simulink model "sistema_fisico_completo"  (R2023b)
settings: Solver=FixedStepAuto  StartTime=0.0  StopTime=10.0  FixedStep=0.001  RelTol=1e-3
settings Model: Creator=Ferran  LastModifiedBy=Ferran
settings DebuggingCC: AlgebraicLoopMsg=none  ArtificialAlgebraicLoopMsg=none
settings ModelReferenceCC: ModelReferenceMinAlgLoopOccurrences=on

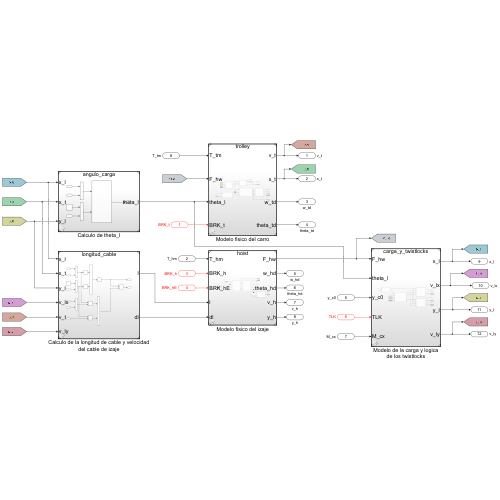
[thumbnail: Simulink's stored preview of the top-level diagram]
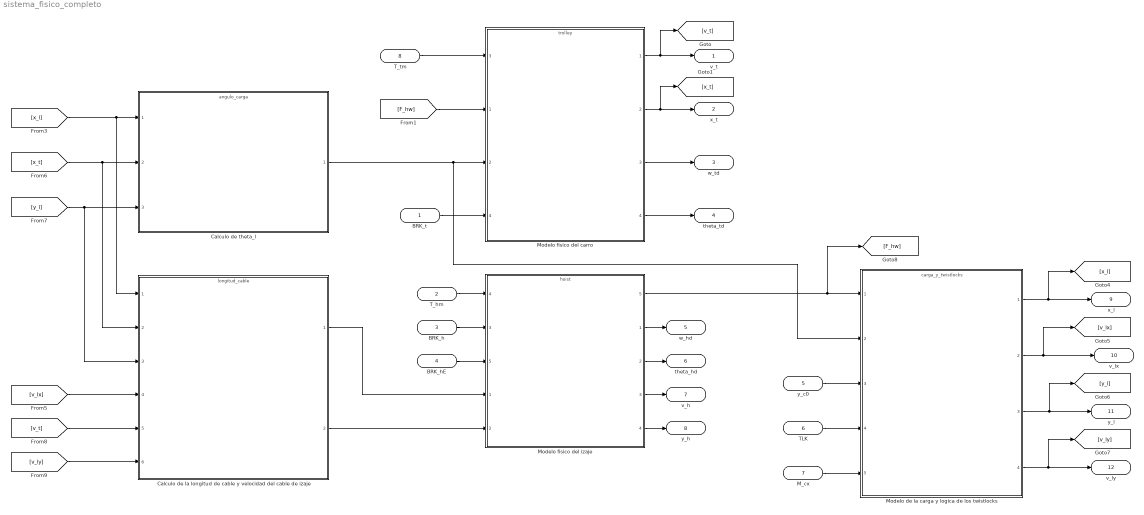
== system sistema_fisico_completo ==
  BRK_t : Inport
  T_hm : Inport  Port=2
  BRK_h : Inport  Port=3
  BRK_hE : Inport  Port=4
  y_c0 : Inport  Port=5
  TLK : Inport  Port=6
  M_cx : Inport  Port=7
  T_tm : Inport  Port=8
  Calculo de la longitud de cable y velocidad del cable de izaje : ModelReference  ModelNameDialog=longitud_cable.slx  SimulationMode=Normal  ModelReferenceVersion=1.4
  Calculo de theta_l : ModelReference  ModelNameDialog=angulo_carga.slx  SimulationMode=Normal  ModelReferenceVersion=1.3
  Modelo de la carga y logica de los twistlocks : ModelReference  ModelNameDialog=carga_y_twistlocks.slx  SimulationMode=Normal  ModelReferenceVersion=1.14
  Modelo fisico del carro : ModelReference  ModelNameDialog=trolley.slx  SimulationMode=Normal  ModelReferenceVersion=1.27
      settings: PortSchema="{\"entries\":[{\"content\":{\"sides\":[{\"content\":{\"connectorIds\":[\"In3\",\"In1\",\"In2\",\"In4\"]},\"type\":\"ConnectorPlacement.EquallySpacedRectSide\",\"uuid\":\"38a31379-7a02-4531-af9b-82f32436a2ed\"},{\"content\":{\"connectorIds\":[\"Out1\",\"Out2\",\"Out3\",\"Out4\"],\"side\":\"RIGHT\"},\"type\":\"ConnectorPlacement.EquallySpacedRectSide\",\"uuid\":\"953f32c8-509d-4a74-a27c-0c30002e5aa6\"},{\"content\":{\"side\":\"TOP\"},\"type\":\"ConnectorPlacement.EquallySpacedRectSide\",\"uuid\":\"64fb0ed3-f874-48da-a9ca-0df566987d1c\"}]},\"type\":\"ConnectorPlacement.EquallySpacedConnector\",\"uuid\":\"ea4c7909-5c74-4284-a576-3672d22ceffd\"}],\"packageUris\":[\"http://schema.mathworks.com/mf0/Connector/R2020b\"],\"version\":\"1.0\"}"
  Modelo fisico del izaje : ModelReference  ModelNameDialog=hoist.slx  SimulationMode=Normal  ModelReferenceVersion=1.22
      settings: PortSchema="{\"entries\":[{\"content\":{\"sides\":[{\"content\":{\"connectorIds\":[\"In4\",\"In3\",\"In5\",\"In1\",\"In2\"]},\"type\":\"ConnectorPlacement.EquallySpacedRectSide\",\"uuid\":\"17f6338c-3c51-40de-9973-080572c91603\"},{\"content\":{\"connectorIds\":[\"Out5\",\"Out1\",\"Out2\",\"Out3\",\"Out4\"],\"side\":\"RIGHT\"},\"type\":\"ConnectorPlacement.EquallySpacedRectSide\",\"uuid\":\"7e968b16-4cea-43bb-a5ca-e4df3289f40a\"},{\"content\":{\"side\":\"TOP\"},\"type\":\"ConnectorPlacement.EquallySpacedRectSide\",\"uuid\":\"93c8c357-b571-41b6-8c5b-1c91e217cb64\"}]},\"type\":\"ConnectorPlacement.EquallySpacedConnector\",\"uuid\":\"e66d9c43-4482-4d93-9c83-496ca9c2d477\"}],\"packageUris\":[\"http://schema.mathworks.com/mf0/Connector/R2020b\"],\"version\":\"1.0\"}"
  v_t : Outport
  x_t : Outport  Port=2
  w_td : Outport  Port=3
  theta_td : Outport  Port=4
  w_hd : Outport  Port=5
  theta_hd : Outport  Port=6
  v_h : Outport  Port=7
  y_h : Outport  Port=8
  x_l : Outport  Port=9
  v_lx : Outport  Port=10
  y_l : Outport  Port=11
  v_ly : Outport  Port=12
  wires:
  Calculo de la longitud de cable y velocidad del cable de izaje/1 -> Modelo fisico del izaje/1
  Calculo de la longitud de cable y velocidad del cable de izaje/2 -> Modelo fisico del izaje/2
  Calculo de theta_l/1 -> Modelo fisico del carro/2, Modelo de la carga y logica de los twistlocks/2
  T_tm/1 -> Modelo fisico del carro/3
  BRK_t/1 -> Modelo fisico del carro/4
  T_hm/1 -> Modelo fisico del izaje/4
  BRK_h/1 -> Modelo fisico del izaje/3
  BRK_hE/1 -> Modelo fisico del izaje/5
  Modelo fisico del izaje/5 -> [F_hw], Modelo de la carga y logica de los twistlocks/1
  y_c0/1 -> Modelo de la carga y logica de los twistlocks/3
  TLK/1 -> Modelo de la carga y logica de los twistlocks/4
  M_cx/1 -> Modelo de la carga y logica de los twistlocks/5
  Modelo fisico del carro/1 -> [v_t], v_t/1
  Modelo fisico del carro/2 -> x_t/1, [x_t]
  Modelo fisico del carro/3 -> w_td/1
  Modelo fisico del carro/4 -> theta_td/1
  Modelo de la carga y logica de los twistlocks/1 -> x_l/1, [x_l]
  Modelo de la carga y logica de los twistlocks/2 -> v_lx/1, [v_lx]
  Modelo de la carga y logica de los twistlocks/3 -> y_l/1, [y_l]
  Modelo de la carga y logica de los twistlocks/4 -> v_ly/1, [v_ly]
  [x_l] -> Calculo de theta_l/1, Calculo de la longitud de cable y velocidad del cable de izaje/1
  [y_l] -> Calculo de theta_l/3, Calculo de la longitud de cable y velocidad del cable de izaje/3
  [x_t] -> Calculo de theta_l/2, Calculo de la longitud de cable y velocidad del cable de izaje/2
  [v_lx] -> Calculo de la longitud de cable y velocidad del cable de izaje/4
  [v_t] -> Calculo de la longitud de cable y velocidad del cable de izaje/5
  [v_ly] -> Calculo de la longitud de cable y velocidad del cable de izaje/6
  Modelo fisico del izaje/1 -> w_hd/1
  Modelo fisico del izaje/2 -> theta_hd/1
  Modelo fisico del izaje/3 -> v_h/1
  Modelo fisico del izaje/4 -> y_h/1
  [F_hw] -> Modelo fisico del carro/1
